simulink model "ME486C_Dyno_DAQ_Test_Version"  (R2025a)
settings: Solver=FixedStepDiscrete  StartTime=0.0  StopTime=20.0  FixedStep=0.02  RelTol=1e-3
settings Model: Creator=YHQ  LastModifiedBy=YHQ

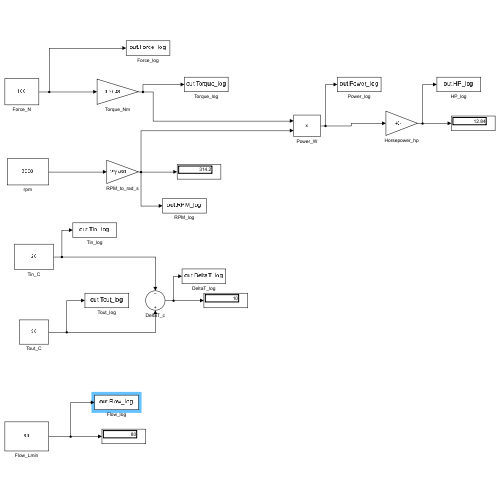
[thumbnail: Simulink's stored preview of the top-level diagram]
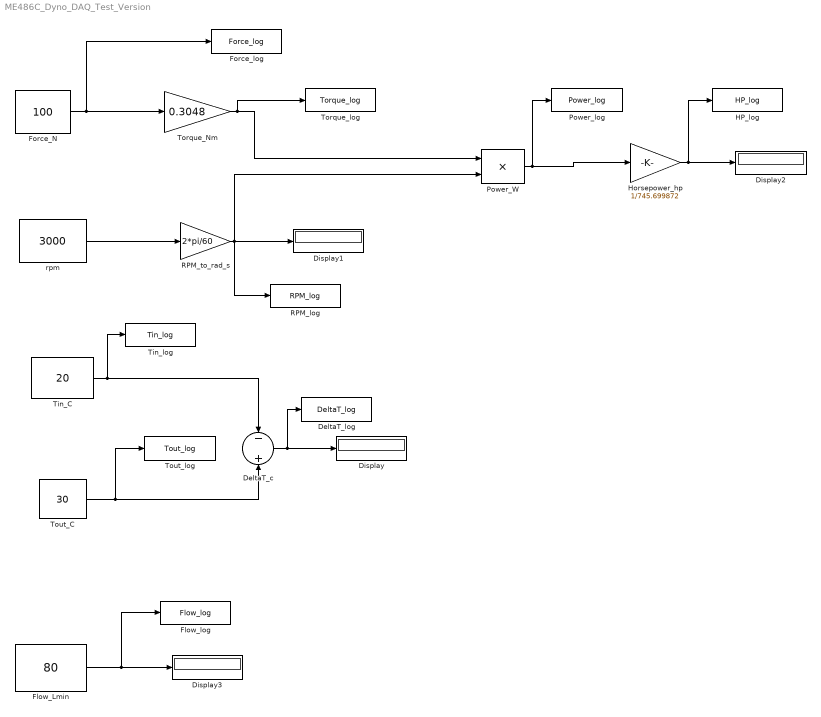
== system ME486C_Dyno_DAQ_Test_Version ==
  DeltaT_c : Sum  Inputs=-+
  DeltaT_log : ToWorkspace  VariableName=DeltaT_log  SaveFormat=Timeseries  SampleTime=-1
  Display{,1..3} (4 alike) : Display
  Flow_Lmin : Constant  Value=80
  Flow_log : ToWorkspace  VariableName=Flow_log  SaveFormat=Timeseries  SampleTime=-1
  Force_N : Constant  Value=100
  Force_log : ToWorkspace  VariableName=Force_log  SaveFormat=Timeseries  SampleTime=-1
  HP_log : ToWorkspace  VariableName=HP_log  SaveFormat=Timeseries  SampleTime=-1
  Horsepower_hp : Gain  Gain=1/745.699872
  Power_W : Product
  Power_log : ToWorkspace  VariableName=Power_log  SaveFormat=Timeseries  SampleTime=-1
  RPM_log : ToWorkspace  VariableName=RPM_log  SaveFormat=Timeseries  SampleTime=-1
  RPM_to_rad_s : Gain  Gain=2*pi/60
  Tin_C : Constant  Value=20
  Tin_log : ToWorkspace  VariableName=Tin_log  SaveFormat=Timeseries  SampleTime=-1
  Torque_Nm : Gain  Gain=0.3048
  Torque_log : ToWorkspace  VariableName=Torque_log  SaveFormat=Timeseries  SampleTime=-1
  Tout_C : Constant  Value=30
  Tout_log : ToWorkspace  VariableName=Tout_log  SaveFormat=Timeseries  SampleTime=-1
  rpm : Constant  Value=3000
  wires:
  Force_N/1 -> Force_log/1, Torque_Nm/1
  rpm/1 -> RPM_to_rad_s/1
  RPM_to_rad_s/1 -> RPM_log/1, Power_W/2, Display1/1
  Torque_Nm/1 -> Torque_log/1, Power_W/1
  Power_W/1 -> Power_log/1, Horsepower_hp/1
  Horsepower_hp/1 -> HP_log/1, Display2/1
  Flow_Lmin/1 -> Flow_log/1, Display3/1
  DeltaT_c/1 -> DeltaT_log/1, Display/1
  Tin_C/1 -> Tin_log/1, DeltaT_c/1
  Tout_C/1 -> Tout_log/1, DeltaT_c/2
